simulink model "testplanner2_cs"  (R2020b)
settings: Solver=ode5  StartTime=0.0  StopTime=30  FixedStep=1/1000  RelTol=1e-3
PreLoadFcn:
  | mbxruntime.callbacks.PreLoadFcn(bdroot);
PostLoadFcn:
  | mbxruntime.callbacks.PostLoadFcn(bdroot);
InitFcn:
  | mbxruntime.callbacks.InitFcn(bdroot);
StartFcn:
  | mbxruntime.callbacks.StartFcn(bdroot);
StopFcn:
  | mbxruntime.callbacks.StopFcn(bdroot);
model workspace (MAT data in the model file):
  mbox_table : object (value not decoded)
  model_closed = 0
  sim_status = 0
values from neighbouring files (symbols this model uses):
  global_path_x = [-6.954 -5.95461774493 -4.95649463442 -3.95964775065 -2.96408287721 -1.96980164192 -0.976804144314 0.0149100776382 1.00534169183 1.99449144113 2.98236009523 3.96894843293 ... (3001 elements, 3001x1)]    [global_path.mat]
  global_path_y = [5.4884 5.4884 5.4884 5.4884 5.4884 5.4884 5.4884 5.4884 5.4884 5.4884 5.4884 5.4884 ... (3001 elements, 3001x1)]    [global_path.mat]
undefined symbols (not defined in the file or in its folder): aubr, c_factor, cf, cr, DiscIntNeverNeededParam, KD_PID_distance, KD_PID_speed, KI_PID_distance, KI_PID_speed, KP_PID_distance, KP_PID_speed, la, lb, LQR_K1, LQR_K2, LQR_K3, LQR_K4, m, rack_displacement, right_wheel_ground, tablebr, vubr, vx_break_point, warningInitialVelocity, x0
libraries: PreScanSimulinkLibrary x51, simulink x19, simulink_extras x11, Solver_SF x1
(part 13 of 13)

== matlab function testplanner2_cs/Audi_A8_Sedan_1/planning module/referenceline provider/MATLAB Function6 ==
  data: x_set input; match_point_index_set output; y_set input; frenet_path_x input; frenet_path_y input; frenet_path_heading input; frenet_path_kappa input; proj_x_set output; proj_y_set output; proj_heading_set output; proj_kappa_set output
function [match_point_index_set,proj_x_set, proj_y_set,proj_heading_set,proj_kappa_set] = ...
    fcn(x_set,y_set,frenet_path_x,frenet_path_y,frenet_path_heading,frenet_path_kappa)
%该函数将批量计算x_set，y_set中的xy，在frenet_path下的投影的信息
%输入 x_set,y_set，待投影的点的集合
%x_set,y_set,frenet_path_x,frenet_path_y,frenet_path_heading,frenet_path_kappa
%曲线在直角坐标系下的x，y，heading，kappa
%输出：match_point_index_set 匹配点在frenet_path下的编号的集合(即从全局路径第一个点开始数，第几个点是匹配点)
%     proj_x y heading kappa 投影的x,y,heading,kappa的集合

% 由于事先不知道x_set中到底有多少个点需要投影，因此事先声明一个最大的数量的点作为缓冲
n = 128;
% 并且由于不知道投影点的个数，所以也不知道输出的个数，因此输出也要做缓冲，用nan表示不存在的点
% 输出最多输出128个
% 输出初始化
match_point_index_set = ones(n,1) * nan;
proj_x_set = ones(n,1) * nan;
proj_y_set = ones(n,1) * nan;
proj_heading_set = ones(n,1) * nan;
proj_kappa_set = ones(n,1) * nan;

% 找匹配点，需要利用上一个周期的结果作为下一个周期遍历的起点，因此需要声明两个全局变量

persistent is_first_run;
persistent pre_match_point_index_set;%bug :pre_match_point_index(i) 未必代表的是第i个障碍物的match_point_index
persistent pre_frenet_path_x;
persistent pre_frenet_path_y;
persistent pre_frenet_path_heading;
persistent pre_frenet_path_kappa;
persistent pre_x_set;
persistent pre_y_set;
%算法主函数入口

if isempty(is_first_run)
    %该if分支表示函数首次运行
    is_first_run = 0;
    pre_frenet_path_x = frenet_path_x;
    pre_frenet_path_y = frenet_path_y;
    pre_frenet_path_heading = frenet_path_heading;
    pre_frenet_path_kappa = frenet_path_kappa;
    %要记录首次运行计算的匹配点的结果供下个周期运行，先初始化
    pre_match_point_index_set = ones(n,1) * nan;
    %对x_set,y_set的点做遍历，找到他们的匹配点
    for i = 1 : length(x_set)
        if isnan(x_set(i))
            break;
        end
        %首次运行时，没有任何提示，只能从frenet path的第一个点开始找
        start_search_index = 1;
        % 声明increase_count，用于表示在遍历时distance连续增加的个数
        increase_count = 0;
        % 开始遍历
        min_distance = inf;
        for j = start_search_index : length(frenet_path_x)
            distance = (x_set(i) - frenet_path_x(j))^2 + (y_set(i) - frenet_path_y(j))^2;
            if distance < min_distance
                min_distance = distance;
                match_point_index_set(i) = j;
                increase_count = 0;
            else
                increase_count = increase_count + 1;
            end
            %如果distance连续增加50次就不要再遍历了，节省时间
            if increase_count > 50
                break;
            end
        end
        
        
        
        %取出匹配点的编号
        match_point_index = match_point_index_set(i);
        %取出匹配点的信息
        match_point_x = frenet_path_x(match_point_index);
        match_point_y = frenet_path_y(match_point_index);
        match_point_heading = frenet_path_heading(match_point_index);
        match_point_kappa = frenet_path_kappa(match_point_index);
        %计算匹配点的方向向量与法向量
        vector_match_point = [match_point_x;match_point_y];
        vector_match_point_direction = [cos(match_point_heading);sin(match_point_heading)];
        %声明待投影点的位矢
        vector_r = [x_set(i);y_set(i)];
        
       %通过匹配点计算投影点
       vector_d = vector_r - vector_match_point;
       ds = vector_d' * vector_match_point_direction;
       vector_proj_point = vector_match_point + ds * vector_match_point_direction;
       proj_heading = match_point_heading + match_point_kappa * ds;
       proj_kappa = match_point_kappa;
       %计算结果输出
       proj_x_set(i) = vector_proj_point(1);
       proj_y_set(i) = vector_proj_point(2);
       proj_heading_set(i) = proj_heading;
       proj_kappa_set(i) = proj_kappa;
    end
    %匹配点的计算结果保存，供下一个周期使用
    pre_match_point_index_set = match_point_index_set;
    pre_x_set = x_set;
    pre_y_set = y_set;
else
    %此if分支表示不是首次运行
    %对每个x_set上的点做处理
    for i = 1 : length(x_set)
        %不是首次运行，对于点x_set(i),y_set(i)来说,start_search_index =
        %pre_match_point_index_set(i)
        start_search_index = pre_match_point_index_set(i);%上个周期匹配点的编号作为本周期搜索的起点
        % 判断帧与帧之间的障碍物是否为同一个
        square_dis = (x_set(i) - pre_x_set(i))^2 + (y_set(i) - pre_y_set(i))^2;
        if square_dis > 36
            % 帧与帧之间的物体的位置距离过大，认为是两个障碍物
            start_search_index = nan;
        end
        % 声明increase_count，用于表示在遍历时distance连续增加的个数
        %%%%%%%%%
        %对于障碍物检测而言，当感知第一次检测到障碍物时，算法并不是首次运行，此时 
        %pre_match_point_index_set的值是nan，如果还用上一时刻的结果作为本周期搜索的起点
        %必然会出问题，所以要修改
        % 声明increase_count_limit
        increase_count_limit = 5;
        if isnan(start_search_index)
            %没有上个周期的结果，那就不能只检查5次了
            increase_count_limit = 50;
            %搜索起点也要设为1
            start_search_index = 1;
        end
        increase_count = 0;
        % 开始遍历
        %这里多一个步骤，判断遍历的方向
        %计算上个周期匹配点的位矢
        vector_pre_match_point = [pre_frenet_path_x(start_search_index);pre_frenet_path_y(start_search_index)];
        vector_pre_match_point_direction = ...
            [cos(pre_frenet_path_heading(start_search_index));sin(pre_frenet_path_heading(start_search_index))];
        %判断遍历的方向
        flag = ([x_set(i);y_set(i)] - vector_pre_match_point)' * vector_pre_match_point_direction;
        min_distance = inf;
        if flag > 0.001
            for j = start_search_index : length(frenet_path_x)
                distance = (x_set(i) - frenet_path_x(j))^2 + (y_set(i) - frenet_path_y(j))^2;
                if distance < min_distance
                    min_distance = distance;
                    match_point_index_set(i) = j;
                    increase_count = 0;
                else
                    increase_count = increase_count + 1;
                end
                %如果distance连续增加increase_count_limit次就不要再遍历了，节省时间
                if increase_count > increase_count_limit
                    break;
                end
            end
        elseif flag < - 0.001
            for j = start_search_index : -1 : 1
                distance = (x_set(i) - frenet_path_x(j))^2 + (y_set(i) - frenet_path_y(j))^2;
                if distance < min_distance
                    min_distance = distance;
                    match_point_index_set(i) = j;
                    increase_count = 0;
                else
                    increase_count = increase_count + 1;
                end
                %如果distance连续增加increase_count_limit次就不要再遍历了，节省时间
                if increase_count > increase_count_limit
                    break;
                end
            end
        else
            match_point_index_set(i) = start_search_index;
        end
        
        %如何通过匹配点计算投影点，请参见《自动驾驶控制算法第七讲》
        %或《自动驾驶决策规划算法》第一章第三节
        
        %取出匹配点的编号
        match_point_index = match_point_index_set(i);
        %取出匹配点的信息
        match_point_x = frenet_path_x(match_point_index);
        match_point_y = frenet_path_y(match_point_index);
        match_point_heading = frenet_path_heading(match_point_index);
        match_point_kappa = frenet_path_kappa(match_point_index);
        %计算匹配点的方向向量与法向量
        vector_match_point = [match_point_x;match_point_y];
        vector_match_point_direction = [cos(match_point_heading);sin(match_point_heading)];
        %声明待投影点的位矢
        vector_r = [x_set(i);y_set(i)];
        
       %通过匹配点计算投影点
       vector_d = vector_r - vector_match_point;
       ds = vector_d' * vector_match_point_direction;
       vector_proj_point = vector_match_point + ds * vector_match_point_direction;
       proj_heading = match_point_heading + match_point_kappa * ds;
       proj_kappa = match_point_kappa;
       %计算结果输出
       proj_x_set(i) = vector_proj_point(1);
       proj_y_set(i) = vector_proj_point(2);
       proj_heading_set(i) = proj_heading;
       proj_kappa_set(i) = proj_kappa;
  
    end
    %匹配点的计算结果保存，供下一个周期使用
    pre_match_point_index_set = match_point_index_set;
    pre_frenet_path_x = frenet_path_x;
    pre_frenet_path_y = frenet_path_y;
    pre_frenet_path_heading = frenet_path_heading;
    pre_frenet_path_kappa = frenet_path_kappa;
    pre_x_set = x_set;
    pre_y_set = y_set;
end

== matlab function testplanner2_cs/Audi_A8_Sedan_1/planning module/EM Planner/Cartesian2Frenet/MATLAB Function2 ==
  data: ax_set input; s_dot2_set output; ay_set input; proj_heading_set input; proj_kappa_set input; l_set input; s_dot_set input; dl_set input; l_dot2_set output; ddl_set output
function [s_dot2_set,l_dot2_set,ddl_set] = fcn(ax_set,ay_set,proj_heading_set,proj_kappa_set,l_set,s_dot_set,dl_set)
%由于不知道有多少个点需要做坐标转换，设一个最大值做缓冲
n = 128;
% 输出初始化
s_dot2_set = ones(n,1)*nan;
l_dot2_set = ones(n,1)*nan;
ddl_set = ones(n,1)*nan;

for i = 1:length(l_set)
    if isnan(l_set(i))
       break;
    end
    a_h = [ax_set(i);ay_set(i)];
    n_r = [-sin(proj_heading_set(i));cos(proj_heading_set(i))];
    t_r = [cos(proj_heading_set(i));sin(proj_heading_set(i))];
    %近似认为dkr/ds 为0 简化计算
    l_dot2_set(i) = a_h'*n_r - proj_kappa_set(i) * (1 - proj_kappa_set(i) * l_set(i)) * s_dot_set(i)^2;
    s_dot2_set(i) = (1/(1 - proj_kappa_set(i) * l_set(i)))* (a_h' * t_r + 2 * proj_kappa_set(i) * dl_set(i) * s_dot_set(i)^2);
    % 要考虑加速度为0的情况
    if (s_dot2_set(i) < 1e-6)
        ddl_set(i) = 0;
    else
        ddl_set(i) = (l_dot2_set(i) - dl_set(i)*s_dot2_set(i))/(s_dot_set(i)^2);
    end
end

== matlab function testplanner2_cs/Audi_A8_Sedan_1/planning module/EM Planner/speed decision with dynamic planning(dp) ==
  data: obs_st_s_in_set input; dp_speed_s output; obs_st_s_out_set input; obs_st_t_in_set input; obs_st_t_out_set input; dp_speed_t output; reference_speed_unlimit input; w_cost_ref_speed input; w_cost_accel input; w_cost_obs input; plan_start_s_dot input
function [dp_speed_s,dp_speed_t] = fcn(obs_st_s_in_set,obs_st_s_out_set,obs_st_t_in_set,obs_st_t_out_set,reference_speed_unlimit...
    ,w_cost_ref_speed,w_cost_accel,w_cost_obs,plan_start_s_dot)
% 速度动态规划
% 时间从0到8开始规划，最多8秒
% s的范围从0开始到路径规划的path的总长度为止
% 为了减少算力 采用非均匀采样，s越小的越密，越大的越稀疏

s_list = [0:0.5:4.5,...
          5.5:1:14.5,...
          16:1.5:29.5,...
          32:2.5:54.5];
% t 采用均匀采样每 0.5s采样一个点
t_list = 0.5:0.5:8;
% 声明st代价矩阵，表示从起点开始到(i,j)点的最小代价为dp_st_cost(i,j)
% s 采样40个 t 采样 16个 一共是 40 * 16
dp_st_cost = ones(40,16) * inf; % 首先初始化为无穷大
% dp_st_s_dot，表示从起点开始到(i,j)点的最优路径的末速度
dp_st_s_dot = zeros(40,16);
% 需要一个矩阵保持最优路径的前一个节点方便回溯
% dp_st_node(i,j) 表示位置为(i,j)的节点中，最优的上一层节点的行号为dp_st_node(i,j)
dp_st_node = zeros(40,16);
% 计算从dp起点到第一列的cost
for i = 1:length(s_list)
    dp_st_cost(i,1) = CalcDpCost(0,0,i,1,obs_st_s_in_set,obs_st_s_out_set,obs_st_t_in_set,obs_st_t_out_set,...
    w_cost_ref_speed,reference_speed_unlimit,w_cost_accel,w_cost_obs,plan_start_s_dot,s_list,t_list,dp_st_s_dot);
    % 计算第一列所有节点的的s_dot，并存储到dp_st_s_dot中
    % 第一列的前一个节点只有起点，起点的s t 都是0
    [s_end,t_end] = CalcSTCoordinate(i,1,s_list,t_list);
    dp_st_s_dot(i,1) = s_end / t_end;
end
% 动态规划主程序
for i = 2:length(t_list)
    % i 为列循环
    for j = 1:length(s_list)
        % j 为行循环
        % 当前行为 j 列为 i
        cur_row = j;
        cur_col = i;
        % 遍历前一列
        for k = 1:length(s_list)
            pre_row = k;
            pre_col = i - 1;
            % 计算边的代价 其中起点为pre_row,pre_col 终点为cur_row cur_col
            cost_temp = CalcDpCost(pre_row,pre_col,cur_row,cur_col,obs_st_s_in_set,obs_st_s_out_set,...
                obs_st_t_in_set,obs_st_t_out_set,w_cost_ref_speed,reference_speed_unlimit,w_cost_accel,w_cost_obs,...
                plan_start_s_dot,s_list,t_list,dp_st_s_dot);
            if cost_temp + dp_st_cost(pre_row,pre_col) < dp_st_cost(cur_row,cur_col)
                dp_st_cost(cur_row,cur_col) = cost_temp + dp_st_cost(pre_row,pre_col);
                % 计算最优的s_dot
                [s_start,t_start] = CalcSTCoordinate(pre_row,pre_col,s_list,t_list);
                [s_end,t_end] = CalcSTCoordinate(cur_row,cur_col,s_list,t_list);
                dp_st_s_dot(cur_row,cur_col) = (s_end - s_start) / (t_end - t_start);
                % 将最短路径的前一个节点的行号记录下来
                dp_st_node(cur_row,cur_col) = pre_row;
            end      
        end
    end
end
% 输出初始化
dp_speed_s = ones(length(t_list),1) * nan;
dp_speed_t = dp_speed_s;
% 找到dp_node_cost 上边界和右边界代价最小的节点
min_cost = inf;
min_row = inf;
min_col = inf;
for i = 1:length(s_list)
    % 遍历右边界
    if dp_st_cost(i,length(t_list)) <= min_cost
        min_cost = dp_st_cost(i,length(t_list));
        min_row = i;
        min_col = length(t_list);
    end
end

for j = 1:length(t_list)
    % 遍历上边界
    if dp_st_cost(1,j) <= min_cost
        min_cost = dp_st_cost(1,j);
        min_row = 1;
        min_col = j;
    end
end
% 这里要注意，虽然我们在t上每0.5s采样一个时间，采了16个点，但是min_col 未必等于16
% 也就是说动态规划的最优解的时间未必是8秒
% 所以我们动态规划最后的输出s t 不一定是写满
% 先把终点的ST输出出来
[dp_speed_s(min_col),dp_speed_t(min_col)] = CalcSTCoordinate(min_row,min_col,s_list,t_list);
% 反向回溯
while min_col ~= 1
    pre_row = dp_st_node(min_row,min_col);
    pre_col = min_col - 1;
    [dp_speed_s(pre_col),dp_speed_t(pre_col)] = CalcSTCoordinate(pre_row,pre_col,s_list,t_list);
    min_row = pre_row;
    min_col = pre_col;
end


end

function cost = CalcDpCost(row_start,col_start,row_end,col_end,obs_st_s_in_set,obs_st_s_out_set,obs_st_t_in_set,obs_st_t_out_set,...
    w_cost_ref_speed,reference_speed,w_cost_accel,w_cost_obs,plan_start_s_dot,s_list,t_list,dp_st_s_dot)
    % 该函数将计算链接两个节点之间边的代价
    % 输入：边的起点的行列号row_start,col_start 边的终点行列号row_end,col_end
          % 障碍物st信息obs_st_s_in_set,obs_st_s_out_set,obs_st_t_in_set,obs_st_t_out_set
          % 推荐速度代价权重w_cost_ref_speed,加速度代价权重w_cost_accel,障碍物代价权重w_cost_obs
          % 推荐速度reference_speed
          % 拼接起点的速度plan_start_s_dot
          % s_list,t_list 采样距离
          % dp_st_s_dot 用于计算加速度
    % 首先计算终点的st坐标
    [s_end,t_end] = CalcSTCoordinate(row_end,col_end,s_list,t_list);
    % 规定起点的行列号为0 
    if row_start == 0
        % 边的起点为dp的起点
        s_start = 0;
        t_start = 0;
        s_dot_start = plan_start_s_dot;
    else
        % 边的起点不是dp的起点
        [s_start,t_start] = CalcSTCoordinate(row_start,col_start,s_list,t_list);
        s_dot_start = dp_st_s_dot(row_start,col_start);
    end
    cur_s_dot = (s_end - s_start) / (t_end - t_start);
    cur_s_dot2 = (cur_s_dot - s_dot_start)/(t_end - t_start);
    % 计算推荐速度代价
    cost_ref_speed = w_cost_ref_speed * (cur_s_dot - reference_speed)^2;
    % 计算加速度代价，这里注意，加速度不能超过车辆动力学上下限
    if cur_s_dot2 < 4 && cur_s_dot2 > -6
        cost_accel = w_cost_accel * cur_s_dot2^2;
    else
        % 超过车辆动力学限制，代价会增大很多倍
        cost_accel = 100000 * w_cost_accel * cur_s_dot2^2;
    end
    cost_obs = CalcObsCost(s_start,t_start,s_end,t_end,obs_st_s_in_set,obs_st_s_out_set,obs_st_t_in_set,obs_st_t_out_set,w_cost_obs);
    cost = cost_obs + cost_accel + cost_ref_speed;
end

function obs_cost = CalcObsCost(s_start,t_start,s_end,t_end,obs_st_s_in_set,obs_st_s_out_set,obs_st_t_in_set,obs_st_t_out_set,w_cost_obs)
% 该函数将计算边的障碍物代价
% 输入：边的起点终点s_start,t_start,s_end,t_end
%       障碍物信息 obs_st_s_in_set,obs_st_s_out_set,obs_st_t_in_set,obs_st_t_out_set
%       障碍物代价权重w_cost_obs
% 输出：边的障碍物代价obs_cost
  % 输出初始化
  obs_cost = 0;
  % 采样点的个数
  n = 5;
  % 采样时间间隔
  dt = (t_end - t_start)/(n - 1);
  % 边的斜率
  k = (s_end - s_start)/(t_end - t_start);
  for i = 1:n
      % 计算采样点的坐标
      t = t_start + (i - 1) * dt;
      s = s_start + k * (i - 1) * dt;
      % 遍历所有障碍物
      for j = 1:length(obs_st_s_in_set)
          if isnan(obs_st_s_in_set(j))
              continue;
          end
          % 计算点到st线段的最短距离
          vector1 = [obs_st_s_in_set(j);obs_st_t_in_set(j)] - [s;t];
          vector2 = [obs_st_s_out_set(j);obs_st_t_out_set(j)] - [s;t];
          vector3 = vector2 - vector1;
          min_dis = 0;
          dis1 = sqrt(vector1'*vector1);
          dis2 = sqrt(vector2'*vector2);
          dis3 = abs(vector1(1)*vector3(2) - vector1(2)*vector3(1))/sqrt(vector3'*vector3);
          if (vector1'*vector3 > 0 && vector2'*vector3 > 0) || (vector1'*vector3 < 0 && vector2'*vector3 < 0)
              min_dis = min(dis1,dis2);
          else
              min_dis = dis3;
          end
          obs_cost = obs_cost + CalcCollisionCost(w_cost_obs,min_dis); 
      end
  end
      
end

function collision_cost = CalcCollisionCost(w_cost_obs,min_dis)
  if abs(min_dis) < 0.5
      collision_cost = w_cost_obs;
  elseif abs(min_dis) > 0.5 && abs(min_dis) < 1.5
      % min_dis = 0.5    collision_cost = w_cost_obs^1;
      % min_dis = 1.5    collision_cost = w_cost_obs^0 = 1
      collision_cost = w_cost_obs^((0.5 - min_dis) + 1);
  else
      collision_cost = 0;
  end
end

function [s_value,t_value] = CalcSTCoordinate(row,col,s_list,t_list)
% 该函数将计算矩阵节点的s t 坐标
% 输入 row col 节点在矩阵的行号和列号
%      s_list t_list 采样间隔表
% 输出：s_value t_value 节点的 s t坐标
% 矩阵的(1,1) 代表的是最左上角的元素 s 最大 t 最小
% * 。。。。。。。。
% * 。。。。。。。。
% * 。。。。。。。。
% * 。。。。。。。。
% *****************

% 首先取出矩阵的行数
m = length(s_list);
% 1 1 对应的是 s 的最大值 t 的最小值
s_value = s_list(m - row + 1);
t_value = t_list(col);
end

== matlab function testplanner2_cs/Audi_A8_Sedan_1/planning module/EM Planner/generate convex space ==
  data: dp_speed_s input; s_lb output; dp_speed_t input; path_index2s input; obs_st_s_in_set input; obs_st_s_out_set input; obs_st_t_in_set input; obs_st_t_out_set input; s_ub output; s_dot_lb output; s_dot_ub output; trajectory_kappa_init input; max_lateral_accel input
function [s_lb,s_ub,s_dot_lb,s_dot_ub] = fcn(dp_speed_s,dp_speed_t,path_index2s,obs_st_s_in_set,obs_st_s_out_set,...
    obs_st_t_in_set,obs_st_t_out_set,trajectory_kappa_init,max_lateral_accel)
% 该函数将计算出s,s_dot的上下界，开辟凸空间供二次规划使用
% dp_speed_s t 最多有16个，输出初始化n = 16
n = 16;
s_lb = ones(n,1)*-inf;
s_ub = ones(n,1)*inf;
s_dot_lb = ones(n,1)*-inf;
s_dot_ub = ones(n,1)*inf;
path_index2s_end_index = length(path_index2s);
dp_speed_end_index = length(dp_speed_s);

% path_index2s也是有缓冲的，找到有效的path_index2s的末尾的位置，赋值给path_index2s_end_index
for k = 2:length(path_index2s)
    if path_index2s(k) == 0 && path_index2s(k-1) ~= 0
        path_index2s_end_index = k - 1;
        break;
    end
    path_index2s_end_index = k;
end
% 找到dp_speed_s中有效的位置，赋值给dp_speed_end_index
for k = 1:length(dp_speed_s)
    if isnan(dp_speed_s(k))
        dp_speed_end_index = k - 1;
        break;
    end
end

for i = 1:n
    % 该循环将施加车辆动力学约束
    if isnan(dp_speed_s(i))
        break;
    end
    cur_s = dp_speed_s(i);
    % 通过插值的方式找到cur_s 所对应的曲率
    cur_kappa = interp1(path_index2s(1:path_index2s_end_index),trajectory_kappa_init(1:path_index2s_end_index),cur_s);
    % a = v^2 * k => v^2 = a/k 注意除0保护
    max_speed =  sqrt(max_lateral_accel / (abs(cur_kappa) + 1e-10));
    min_speed = 0;
    s_dot_lb(i) = min_speed;
    s_dot_ub(i) = max_speed;    
end



for i = 1:length(obs_st_s_in_set)
    if isnan(obs_st_s_in_set(i))
        continue;
    end
    % 取s t 直线的中点，作为obs_s obs_t 的坐标 
    obs_t = (obs_st_t_in_set(i) + obs_st_t_out_set(i)) / 2;
    obs_s = (obs_st_s_in_set(i) + obs_st_s_out_set(i)) / 2;
    % 计算障碍物的纵向速度
    obs_speed = (obs_st_s_out_set(i) - obs_st_s_in_set(i)) / (obs_st_t_out_set(i) - obs_st_t_in_set(i));
    % 插值找到当t = obs_t时，dp_speed_s 的值
    dp_s = interp1([0;dp_speed_t(1:dp_speed_end_index)],[0;dp_speed_s(1:dp_speed_end_index)],obs_t);
    % 找到dp_speed_t中 与obs_st_t_in_set(i)最近的时间，并将此时间的编号赋值给t_lb_index
    for j = 1:length(dp_speed_t) - 1
        if dp_speed_t(1) > obs_st_t_in_set(i)
            % 如果障碍物切入时间比0.5秒还要短，那么t_lb_index = 1
            break;
        elseif dp_speed_t(j) <= obs_st_t_in_set(i) && dp_speed_t(j + 1) > obs_st_t_in_set(i)
            % 否则遍历dp_speed_t 找到与obs_st_t_in_set(i)最近的点的编号
            break;
        end
    end
    t_lb_index = j;% 将点的编号赋值给j
     % 找到dp_speed_t中 与obs_st_t_out_set(i)最近的时间，并将此时间的编号赋值给t_ub_index
    for j = 1:length(dp_speed_t) - 1
        if dp_speed_t(1) > obs_st_t_out_set(i)
            break;
        elseif dp_speed_t(j) <= obs_st_t_out_set(i) && dp_speed_t(j + 1) > obs_st_t_out_set(i)
            break;
        end
    end
    t_ub_index = j;
    % 这里稍微做个缓冲，把 t_lb_index 稍微缩小一些，t_ub_index稍微放大一些
    t_lb_index = max(t_lb_index - 2,3);% 最低为3 因为碰瓷没法处理
    t_ub_index = min(t_ub_index + 2,dp_speed_end_index);
    if obs_s > dp_s
        % 决策为减速避让
        for m = t_lb_index:t_ub_index
            % 在t_lb_index:t_ub_index的区间上 s的上界不可以超过障碍物st斜直线
            dp_t = dp_speed_t(m);
            s_ub(m) = min(s_ub(m),obs_st_s_in_set(i) + obs_speed * (dp_t - obs_st_t_in_set(i)));
        end
    else 
        % 决策为加速超车
        for m = t_lb_index:t_ub_index
             % 在t_lb_index:t_ub_index的区间上 s的下界不能小于障碍物st斜直线
            dp_t = dp_speed_t(m);
            s_lb(m) = max(s_lb(m),obs_st_s_in_set(i) + obs_speed * (dp_t - obs_st_t_in_set(i)));
        end
    end
        
end

== matlab function testplanner2_cs/Audi_A8_Sedan_1/planning module/EM Planner/MATLAB Function5 ==
  data: dp_speed_s input; dp_speed_t input; qp_speed_s input; qp_speed_t input; obs_s_in_set input; obs_s_out_set input; obs_t_in_set input; obs_t_out_set input
function  fcn(dp_speed_s,dp_speed_t,qp_speed_s,qp_speed_t,obs_s_in_set,obs_s_out_set,obs_t_in_set,obs_t_out_set)
coder.extrinsic("plot");
cla;
n = length(dp_speed_s);
m = length(obs_s_in_set);
s = length(qp_speed_s);
for i = 1:length(dp_speed_s)
    if isnan(dp_speed_s(i))
        n = i -1;
        break;
    end
end
for i = 1:length(qp_speed_s)
    if isnan(qp_speed_s(i))
        s = i -1;
        break;
    end
end

plot(dp_speed_t(1:n),dp_speed_s(1:n),'r')
plot(qp_speed_t(1:s),qp_speed_s(1:s),'b')
hold on
axis([-1 10 -10 50]);
for i = 1:m
    if isnan(obs_s_in_set(i))
        continue;
    end
    point_t = [obs_t_in_set(i),obs_t_out_set(i)];
    point_s = [obs_s_in_set(i),obs_s_out_set(i)];
    plot(point_t,point_s)
end

== matlab function testplanner2_cs/Audi_A8_Sedan_1/planning module/EM Planner/spee planning with quadratic programming (qp) ==
  data: plan_start_s_dot input; qp_s_init output; plan_start_s_dot2 input; dp_speed_s input; dp_speed_t input; s_lb input; s_ub input; s_dot_lb input; s_dot_ub input; qp_s_dot_init output; qp_s_dot2_init output; relative_time_init output; w_cost_s_dot2 input; w_cost_v_ref input; w_cost_jerk input; speed_reference input
function [qp_s_init,qp_s_dot_init,qp_s_dot2_init,relative_time_init] = fcn(plan_start_s_dot,...
    plan_start_s_dot2,dp_speed_s,dp_speed_t,s_lb,s_ub,s_dot_lb,s_dot_ub,w_cost_s_dot2,w_cost_v_ref,w_cost_jerk,speed_reference)
%速度二次规划
% 输入：规划起点plan_start_s_dot,plan_start_s_dot2
%       动态规划结果dp_speed_s,dp_speed_t
%       凸空间约束 s_lb,s_ub,s_dot_lb,s_dot_ub
%       加速度代价权重，推荐速度代价权重，jerk代价权重w_cost_s_dot2,w_cost_v_ref,w_cost_jerk
%       参考速度speed_reference
% 输出：速度曲线qp_s_init,qp_s_dot_init,qp_s_dot2_init,relative_time_init
coder.extrinsic("quadprog")
% 由于dp的结果未必是16，该算法将计算dp_speed_end到底是多少
dp_speed_end = 16;
for i = 1:length(dp_speed_s)
    
    if isnan(dp_speed_s(i))
        dp_speed_end = i - 1;
        break;
    end
end
% 由于dp_speed_end实际上是不确定的，但是输出要求必须是确定长度的值，因此
% 输出初始化选择dp_speed_end的最大值 + 规划起点作为输出初始化的规模
n = 17;

qp_s_init = ones(n,1) * nan;
qp_s_dot_init = ones(n,1) * nan;
qp_s_dot2_init = ones(n,1) * nan;
relative_time_init = ones(n,1) * nan;
s_end = dp_speed_s(dp_speed_end);
% 此时dp_speed_end表示真正有效的dp_speed_t的元素个数，取出dp_speed_t有效的最后一个元素作为规划的时间终点
% 记为recommend_T
recommend_T = dp_speed_t(dp_speed_end);
% qp的规模应该是dp的有效元素的个数 + 规划起点
qp_size = dp_speed_end + 1;
% 连续性约束矩阵初始化，这里的等式约束应该是 Aeq'*X == beq 有转置
Aeq = zeros(3*qp_size,2*qp_size - 2);
beq = zeros(2*qp_size - 2,1);
% 不等式约束初始化
lb = ones(3*qp_size,1);
ub = lb;
% 计算采样间隔时间dt
dt = recommend_T/dp_speed_end;
A_sub =[1,0;
        dt,1;
        (1/3)*dt^2,(1/2)*dt;
        -1,0;
        0,-1;
        (1/6)*dt^2,dt/2];
for i = 1:qp_size - 1
    Aeq(3*i-2:3*i+3,2*i-1:2*i) = A_sub;
end
% 这里初始化不允许倒车约束，也就是 s(i) - s(i+1) <= 0
A = zeros(qp_size-1,3*qp_size);
b = zeros(qp_size-1,1);
for i = 1:qp_size-1
    A(i,3*i - 2) = 1;
    A(i,3*i + 1) = -1;
end
% 由于生成的凸空间约束s_lb s_ub不带起点，所以lb(i) = s_lb(i-1) 以此类推
% 允许最小加速度为-6 最大加速度为4(基于车辆动力学)
for i = 2:qp_size
   lb(3*i - 2) = s_lb(i-1);
   lb(3*i - 1) = s_dot_lb(i-1);
   lb(3*i) = -6;
   ub(3*i - 2) = s_ub(i-1);
   ub(3*i - 1) = s_dot_ub(i-1);
   ub(3*i) = 4;
end
% 起点约束
lb(1) = 0;
lb(2) = plan_start_s_dot;
lb(3) = plan_start_s_dot2;
ub(1) = lb(1);
ub(2) = lb(2);
ub(3) = lb(3);
% 加速度代价 jerk代价 以及推荐速度代价
A_s_dot2 = zeros(3*qp_size,3*qp_size);
A_jerk = zeros(3*qp_size,qp_size - 1);
A_ref = zeros(3*qp_size,3*qp_size);

A4_sub =[0;0;1;0;0;-1];
for i = 1:qp_size
    A_s_dot2(3*i,3*i) = 1;
    A_ref(3*i-1,3*i-1) = 1;
end
for i = 1:qp_size - 1   
   A_jerk(3*i-2:3*i+3,i:i) = A4_sub;
end
% 生成H f
H = w_cost_s_dot2 * (A_s_dot2 * A_s_dot2') + w_cost_jerk * (A_jerk * A_jerk') + w_cost_v_ref * (A_ref * A_ref');
H = 2*H;
f = zeros(3*qp_size,1);
for i = 1:qp_size
    f(3*i-1) =  - 2 * w_cost_v_ref * speed_reference;
end
% 计算二次规划
X = quadprog(H,f,A,b,Aeq',beq,lb,ub);
% 将结果输出
for i = 1:qp_size
   qp_s_init(i) = X(3*i - 2);
   qp_s_dot_init(i) = X(3*i - 1);
   qp_s_dot2_init(i) = X(3*i);
   relative_time_init(i) = (i - 1)*dt;
end

== matlab function testplanner2_cs/Audi_A8_Sedan_2/PathFollower_Preview_1/LateralController/CTRL REFERENCES/Find Reference Point (pref0) on Trajectory closest to P0 Point (p0)/eml_find_closest_trajectory_points0 ==
  data: pvp input size=2; Actor_traj_distance output; TrajOffset_x_y_Y input size=3; ActorOffset_Left_Right input; p0 input size=3; Traj_x parameter; Traj_y parameter; Actor_traj_angle output; RefreshCounter parameter
function [Actor_traj_distance,Actor_traj_angle]  = eml_find_closest_trajectory_points0(pvp,TrajOffset_x_y_Y,ActorOffset_Left_Right,p0,Traj_x,Traj_y,RefreshCounter)

[Actor_traj_distance,Actor_traj_angle]  = emlfcn_find_closest_trajectory_points0(pvp,TrajOffset_x_y_Y,ActorOffset_Left_Right,p0,Traj_x,Traj_y,RefreshCounter);

% end function
